simulink model "plateforme_seule_matlab"  (R2016a)
settings: Solver=VariableStepAuto  StartTime=0.0  StopTime=10  RelTol=1e-3
model workspace: external: MATLAB File C:\Users\costa\Documents\Renaud\Dorian\Prepa\Studies\Carte aquisition Stewart\Matlab-SW\plateforme_seule_matlab_DataFile.m (data not in the file)
values from neighbouring files (symbols this model uses):
  K = 0.0135    [variables.m]
  Kd = 0    [variables.m]
  Ki = 0    [variables.m]
  Kp = 40    [variables.m]
  L0 = 380    [variables.m]
  R = 8.9    [variables.m]
undefined symbols (not defined in the file or in its folder): smiData, X, Y, Z
libraries: sm_lib x361, fl_lib x60, nesl_utility x13, simulink x6
(part 3 of 9)

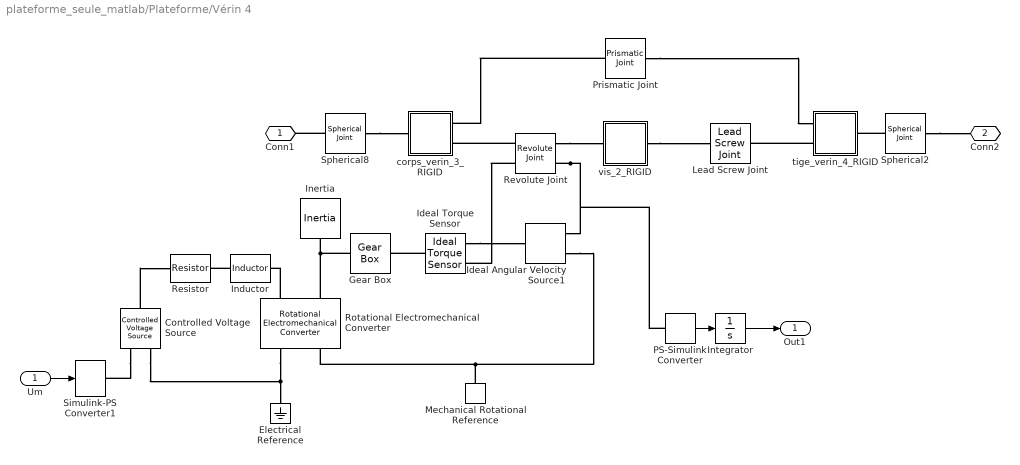
== system plateforme_seule_matlab/Plateforme/Vérin 4 ==
  Um : Inport
  Controlled Voltage Source : fl_lib/Electrical/Electrical Sources/Controlled Voltage Source
  Electrical Reference : fl_lib/Electrical/Electrical Elements/Electrical Reference
  Gear Box : fl_lib/Mechanical/Mechanisms/Gear Box  ratio=red  t_in_specify=off  t_in_priority=None  t_in=0 N*m  t_out_specify=off  t_out_priority=None  t_out=0 N*m
  Ideal Angular Velocity Source1 : fl_lib/Mechanical/Mechanical Sources/Ideal Angular Velocity Source
  Ideal Torque Sensor : fl_lib/Mechanical/Mechanical Sensors/Ideal Torque Sensor
  Inductor : fl_lib/Electrical/Electrical Elements/Inductor  l=L H  r=0 Ohm  g=1e-9 1/Ohm  i_specify=off  i_priority=None  i=0 A  v_specify=off  v_priority=None  v=0 V  i_L_specify=off  i_L_priority=High  i_L=0 A
  Inertia : fl_lib/Mechanical/Rotational Elements/Inertia  inertia=J kg*m^2  w_specify=off  w_priority=High  w=0 rad/s  t_specify=off  t_priority=None  t=0 N*m
  Integrator : Integrator  InitialCondition=L0
  Lead Screw Joint : sm_lib/Joints/Lead Screw Joint  SenseConstraintForce=off  SenseConstraintForceX=off  SenseConstraintForceY=off  SenseConstraintForceZ=off  SenseConstraintTorque=off  SenseConstraintTorqueX=off  SenseConstraintTorqueY=off  SenseConstraintTorqueZ=off  SenseTotalForce=off  SenseTotalForceX=off  SenseTotalForceY=off  SenseTotalForceZ=off  SenseTotalTorque=off  SenseTotalTorqueX=off  SenseTotalTorqueY=off  SenseTotalTorqueZ=off  CompositeWrenchDir=FollowerOnBase  CompositeWrenchFrame=BaseFrame  Direction=RightHand  Lead=6.35  LeadUnits=mm/rev  SenseRotationPosition=off  SenseRotationVelocity=off  SenseRotationAcceleration=off  SenseTranslationPosition=off  SenseTranslationVelocity=off  SenseTranslationAcceleration=off  PositionTargetSpecify=off  PositionTargetPriority=High  PositionTargetRotationBased=off  PositionTargetRotationValue=0  PositionTargetRotationValueUnits=deg  PositionTargetTranslationValue=0  PositionTargetTranslationValueUnits=m  VelocityTargetSpecify=off  VelocityTargetPriority=High  VelocityTargetRotationBased=off  VelocityTargetRotationValue=0  VelocityTargetRotationValueUnits=deg/s  VelocityTargetTranslationValue=0  VelocityTargetTranslationValueUnits=m/s
  Mechanical Rotational Reference : fl_lib/Mechanical/Rotational Elements/Mechanical Rotational Reference
  PS-Simulink Converter : nesl_utility/PS-Simulink Converter  PhysicalDomain=network_engine_domain  SubClassName=ps_output  LeftPortType=input  RightPortType=output  PseudoPeriodic=off  Frequencies=[]  Unit=rad/s  AffineConversion=off
  Prismatic Joint : sm_lib/Joints/Prismatic Joint  SenseConstraintForce=off  SenseConstraintForceX=off  SenseConstraintForceY=off  SenseConstraintForceZ=off  SenseConstraintTorque=off  SenseConstraintTorqueX=off  SenseConstraintTorqueY=off  SenseConstraintTorqueZ=off  SenseTotalForce=off  SenseTotalForceX=off  SenseTotalForceY=off  SenseTotalForceZ=off  SenseTotalTorque=off  SenseTotalTorqueX=off  SenseTotalTorqueY=off  SenseTotalTorqueZ=off  CompositeWrenchDir=FollowerOnBase  CompositeWrenchFrame=BaseFrame  EquilibriumPosition=L0  EquilibriumPositionUnits=m  SpringStiffness=0  SpringStiffnessUnits=N/m  DampingCoefficient=0  DampingCoefficientUnits=N/(m/s)  TorqueActuationMode=NoTorque  MotionActuationMode=ComputedMotion  SensePosition=off  SenseVelocity=off  SenseAcceleration=off  SenseTorqueForce=off  PositionTargetSpecify=off  PositionTargetPriority=High  PositionTargetValue=L0  PositionTargetValueUnits=m  VelocityTargetSpecify=off  VelocityTargetPriority=High  VelocityTargetValue=0  VelocityTargetValueUnits=m/s
  Resistor : fl_lib/Electrical/Electrical Elements/Resistor  R=R Ohm  i_specify=off  i_priority=None  i=0 A  v_specify=off  v_priority=None  v=0 V
  Revolute Joint : sm_lib/Joints/Revolute Joint  SenseConstraintForce=off  SenseConstraintForceX=off  SenseConstraintForceY=off  SenseConstraintForceZ=off  SenseConstraintTorque=off  SenseConstraintTorqueX=off  SenseConstraintTorqueY=off  SenseConstraintTorqueZ=off  SenseTotalForce=off  SenseTotalForceX=off  SenseTotalForceY=off  SenseTotalForceZ=off  SenseTotalTorque=off  SenseTotalTorqueX=off  SenseTotalTorqueY=off  SenseTotalTorqueZ=off  CompositeWrenchDir=FollowerOnBase  CompositeWrenchFrame=BaseFrame  EquilibriumPosition=0  EquilibriumPositionUnits=deg  SpringStiffness=0  SpringStiffnessUnits=N*m/deg  DampingCoefficient=0  DampingCoefficientUnits=N*m/(deg/s)  TorqueActuationMode=InputTorque  MotionActuationMode=ComputedMotion  SensePosition=off  SenseVelocity=on  SenseAcceleration=off  SenseTorqueForce=off  PositionTargetSpecify=off  PositionTargetPriority=High  PositionTargetValue=0  PositionTargetValueUnits=deg  VelocityTargetSpecify=off  VelocityTargetPriority=High  VelocityTargetValue=0  VelocityTargetValueUnits=deg/s
  Rotational Electromechanical Converter : fl_lib/Electrical/Electrical Elements/Rotational Electromechanical Converter  K=K V/(rad/s)  i_specify=off  i_priority=None  i=0 A  v_specify=off  v_priority=None  v=0 V  t_specify=off  t_priority=None  t=0 N*m  w_specify=off  w_priority=None  w=0 rad/s
  Simulink-PS Converter1 : nesl_utility/Simulink-PS Converter  PhysicalDomain=network_engine_domain  SubClassName=ps_input  LeftPortType=input  RightPortType=output  PseudoPeriodic=off  Frequencies=[]  NoiseDistribution=none  NoiseParameters=[]  Unit=V  AffineConversion=off  InputFiltering=off  SimscapeFilterOrder=1  InputFilterTimeConstant=0.001  UdotUserProvided=1
  Spherical2 : sm_lib/Joints/Spherical Joint  SenseConstraintForce=off  SenseConstraintForceX=off  SenseConstraintForceY=off  SenseConstraintForceZ=off  SenseConstraintTorque=off  SenseConstraintTorqueX=off  SenseConstraintTorqueY=off  SenseConstraintTorqueZ=off  SenseTotalForce=off  SenseTotalForceX=off  SenseTotalForceY=off  SenseTotalForceZ=off  SenseTotalTorque=off  SenseTotalTorqueX=off  SenseTotalTorqueY=off  SenseTotalTorqueZ=off  CompositeWrenchDir=FollowerOnBase  CompositeWrenchFrame=BaseFrame  DefPosRotationMethod=None  DefPosRotationAngleUnits=deg  DefPosRotationStandardAxis=+Z  DefPosRotationAngle=0.0  DefPosRotationArbitraryAxis=[0 0 1]  DefPosFollAlignAxisA=+X  DefPosBaseAlignAxisA=+Y  DefPosFollAlignAxisB=+Y  DefPosBaseAlignAxisB=+Z  DefPosRotationSequenceAxes=FollowerAxes  DefPosRotationSequence=XYX  DefPosRotationSequenceAngles=[0 0 0]  DefPosRotationSequenceAnglesUnits=deg  DefPosRotationMatrix=[1 0 0; 0 1 0; 0 0 1]  EqPosRotationMethod=None  EqPosRotationAngleUnits=deg  EqPosRotationStandardAxis=+Z  EqPosRotationAngle=0.0  EqPosRotationArbitraryAxis=[0 0 1]  EqPosFollAlignAxisA=+X  EqPosBaseAlignAxisA=+Y  EqPosFollAlignAxisB=+Y  EqPosBaseAlignAxisB=+Z  EqPosRotationSequenceAxes=FollowerAxes  EqPosRotationSequence=XYX  EqPosRotationSequenceAngles=[0 0 0]  EqPosRotationSequenceAnglesUnits=deg  EqPosRotationMatrix=[1 0 0; 0 1 0; 0 0 1]  SpringStiffness=0  SpringStiffnessUnits=m*N/rad  DampingCoefficient=0  DampingCoefficientUnits=m*s*N/rad  ActuateTorqueX=off  ActuateTorqueY=off  ActuateTorqueZ=off  ActuateTorque=off  TorqueActuationMode=NoTorque  MotionActuationMode=ComputedMotion  ActuationFrame=BaseFrame  SensePosition=off  SenseVelocityX=off  SenseVelocityY=off  SenseVelocityZ=off  SenseVelocity=off  SenseAccelerationX=off  SenseAccelerationY=off  SenseAccelerationZ=off  SenseAcceleration=off  SenseTorqueX=off  SenseTorqueY=off  SenseTorqueZ=off  SenseTorqueForce=off  SensingFrame=FollowerFrame  PositionTargetRotationMethod=None  PositionTargetRotationAngleUnits=deg  PositionTargetRotationStandardAxis=+Z  PositionTargetRotationAngle=0.0  PositionTargetRotationArbitraryAxis=[0 0 1]  PositionTargetFollAlignAxisA=+X  PositionTargetBaseAlignAxisA=+Y  PositionTargetFollAlignAxisB=+Y  PositionTargetBaseAlignAxisB=+Z  PositionTargetRotationSequenceAxes=FollowerAxes  PositionTargetRotationSequence=XYX  PositionTargetRotationSequenceAngles=[0 0 0]  PositionTargetRotationSequenceAnglesUnits=deg  PositionTargetRotationMatrix=[1 0 0; 0 1 0; 0 0 1]  PositionTargetSpecify=off  PositionTargetPriority=High  VelocityTargetValue=[0 0 0]  VelocityTargetValueUnits=deg/s  VelocityTargetSpecify=off  VelocityTargetPriority=High  VelocityTargetInFollowerFrame=on
  Spherical8 : sm_lib/Joints/Spherical Joint  SenseConstraintForce=off  SenseConstraintForceX=off  SenseConstraintForceY=off  SenseConstraintForceZ=off  SenseConstraintTorque=off  SenseConstraintTorqueX=off  SenseConstraintTorqueY=off  SenseConstraintTorqueZ=off  SenseTotalForce=off  SenseTotalForceX=off  SenseTotalForceY=off  SenseTotalForceZ=off  SenseTotalTorque=off  SenseTotalTorqueX=off  SenseTotalTorqueY=off  SenseTotalTorqueZ=off  CompositeWrenchDir=FollowerOnBase  CompositeWrenchFrame=BaseFrame  DefPosRotationMethod=None  DefPosRotationAngleUnits=deg  DefPosRotationStandardAxis=+Z  DefPosRotationAngle=0.0  DefPosRotationArbitraryAxis=[0 0 1]  DefPosFollAlignAxisA=+X  DefPosBaseAlignAxisA=+Y  DefPosFollAlignAxisB=+Y  DefPosBaseAlignAxisB=+Z  DefPosRotationSequenceAxes=FollowerAxes  DefPosRotationSequence=XYX  DefPosRotationSequenceAngles=[0 0 0]  DefPosRotationSequenceAnglesUnits=deg  DefPosRotationMatrix=[1 0 0; 0 1 0; 0 0 1]  EqPosRotationMethod=None  EqPosRotationAngleUnits=deg  EqPosRotationStandardAxis=+Z  EqPosRotationAngle=0.0  EqPosRotationArbitraryAxis=[0 0 1]  EqPosFollAlignAxisA=+X  EqPosBaseAlignAxisA=+Y  EqPosFollAlignAxisB=+Y  EqPosBaseAlignAxisB=+Z  EqPosRotationSequenceAxes=FollowerAxes  EqPosRotationSequence=XYX  EqPosRotationSequenceAngles=[0 0 0]  EqPosRotationSequenceAnglesUnits=deg  EqPosRotationMatrix=[1 0 0; 0 1 0; 0 0 1]  SpringStiffness=0  SpringStiffnessUnits=m*N/rad  DampingCoefficient=0  DampingCoefficientUnits=m*s*N/rad  ActuateTorqueX=off  ActuateTorqueY=off  ActuateTorqueZ=off  ActuateTorque=off  TorqueActuationMode=NoTorque  MotionActuationMode=ComputedMotion  ActuationFrame=BaseFrame  SensePosition=off  SenseVelocityX=off  SenseVelocityY=off  SenseVelocityZ=off  SenseVelocity=off  SenseAccelerationX=off  SenseAccelerationY=off  SenseAccelerationZ=off  SenseAcceleration=off  SenseTorqueX=off  SenseTorqueY=off  SenseTorqueZ=off  SenseTorqueForce=off  SensingFrame=FollowerFrame  PositionTargetRotationMethod=ArbitraryAxis  PositionTargetRotationAngleUnits=deg  PositionTargetRotationStandardAxis=+Z  PositionTargetRotationAngle=smiData.SphericalJoint(9).S.Pos.Angle  PositionTargetRotationArbitraryAxis=smiData.SphericalJoint(9).S.Pos.Axis  PositionTargetFollAlignAxisA=+X  PositionTargetBaseAlignAxisA=+Y  PositionTargetFollAlignAxisB=+Y  PositionTargetBaseAlignAxisB=+Z  PositionTargetRotationSequenceAxes=FollowerAxes  PositionTargetRotationSequence=XYX  PositionTargetRotationSequenceAngles=[0 0 0]  PositionTargetRotationSequenceAnglesUnits=deg  PositionTargetRotationMatrix=[1 0 0; 0 1 0; 0 0 1]  PositionTargetSpecify=off  PositionTargetPriority=Low  VelocityTargetValue=[0 0 0]  VelocityTargetValueUnits=deg/s  VelocityTargetSpecify=off  VelocityTargetPriority=High  VelocityTargetInFollowerFrame=on
  corps_verin_3_RIGID : Subsystem
  tige_verin_4_RIGID : Subsystem
  vis_2_RIGID : Subsystem
  Conn1 : PMIOPort  Port=1  Side=Left
  Conn2 : PMIOPort  Port=2  Side=Right
  Out1 : Outport
  wires:
  Um/1 -> Simulink-PS Converter1/1
  PS-Simulink Converter/1 -> Integrator/1
  Integrator/1 -> Out1/1
  connections:
  Spherical8/LConn1 -- Conn1/RConn1
  Spherical8/RConn1 -- corps_verin_3_RIGID/LConn1
  Spherical2/LConn1 -- tige_verin_4_RIGID/RConn1
  Spherical2/RConn1 -- Conn2/RConn1
  Prismatic Joint/LConn1 -- corps_verin_3_RIGID/RConn1
  Prismatic Joint/RConn1 -- tige_verin_4_RIGID/LConn1
  Revolute Joint/LConn1 -- corps_verin_3_RIGID/RConn2
  tige_verin_4_RIGID/LConn2 -- Lead Screw Joint/RConn1
  vis_2_RIGID/RConn1 -- Lead Screw Joint/LConn1
  Revolute Joint/RConn1 -- vis_2_RIGID/LConn1
  Ideal Angular Velocity Source1/RConn2 -- Mechanical Rotational Reference/LConn1 -- Rotational Electromechanical Converter/RConn2
  Rotational Electromechanical Converter/LConn2 -- Gear Box/LConn1 -- Inertia/LConn1
  Controlled Voltage Source/RConn2 -- Rotational Electromechanical Converter/RConn1 -- Electrical Reference/LConn1
  Revolute Joint/RConn2 -- PS-Simulink Converter/LConn1 -- Ideal Angular Velocity Source1/RConn1
  Rotational Electromechanical Converter/LConn1 -- Inductor/RConn1
  Inductor/LConn1 -- Resistor/RConn1
  Controlled Voltage Source/LConn1 -- Resistor/LConn1
  Ideal Torque Sensor/RConn1 -- Ideal Angular Velocity Source1/LConn1
  Revolute Joint/LConn2 -- Ideal Torque Sensor/RConn2
  Ideal Torque Sensor/LConn1 -- Gear Box/RConn1
  Controlled Voltage Source/RConn1 -- Simulink-PS Converter1/RConn1

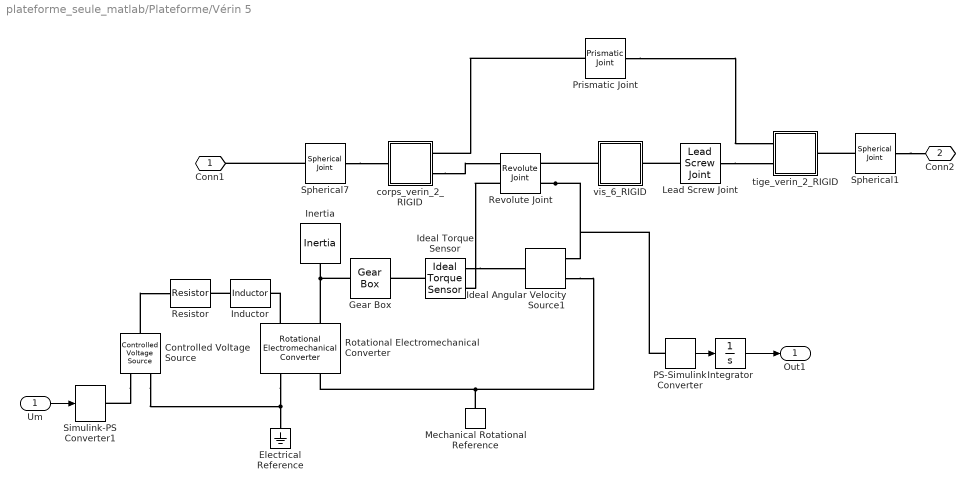
== system plateforme_seule_matlab/Plateforme/Vérin 5 ==
  Um : Inport
  Controlled Voltage Source : fl_lib/Electrical/Electrical Sources/Controlled Voltage Source
  Electrical Reference : fl_lib/Electrical/Electrical Elements/Electrical Reference
  Gear Box : fl_lib/Mechanical/Mechanisms/Gear Box  ratio=red  t_in_specify=off  t_in_priority=None  t_in=0 N*m  t_out_specify=off  t_out_priority=None  t_out=0 N*m
  Ideal Angular Velocity Source1 : fl_lib/Mechanical/Mechanical Sources/Ideal Angular Velocity Source
  Ideal Torque Sensor : fl_lib/Mechanical/Mechanical Sensors/Ideal Torque Sensor
  Inductor : fl_lib/Electrical/Electrical Elements/Inductor  l=L H  r=0 Ohm  g=1e-9 1/Ohm  i_specify=off  i_priority=None  i=0 A  v_specify=off  v_priority=None  v=0 V  i_L_specify=off  i_L_priority=High  i_L=0 A
  Inertia : fl_lib/Mechanical/Rotational Elements/Inertia  inertia=J kg*m^2  w_specify=off  w_priority=High  w=0 rad/s  t_specify=off  t_priority=None  t=0 N*m
  Integrator : Integrator  InitialCondition=L0
  Lead Screw Joint : sm_lib/Joints/Lead Screw Joint  SenseConstraintForce=off  SenseConstraintForceX=off  SenseConstraintForceY=off  SenseConstraintForceZ=off  SenseConstraintTorque=off  SenseConstraintTorqueX=off  SenseConstraintTorqueY=off  SenseConstraintTorqueZ=off  SenseTotalForce=off  SenseTotalForceX=off  SenseTotalForceY=off  SenseTotalForceZ=off  SenseTotalTorque=off  SenseTotalTorqueX=off  SenseTotalTorqueY=off  SenseTotalTorqueZ=off  CompositeWrenchDir=FollowerOnBase  CompositeWrenchFrame=BaseFrame  Direction=RightHand  Lead=6.35  LeadUnits=mm/rev  SenseRotationPosition=off  SenseRotationVelocity=off  SenseRotationAcceleration=off  SenseTranslationPosition=off  SenseTranslationVelocity=off  SenseTranslationAcceleration=off  PositionTargetSpecify=off  PositionTargetPriority=High  PositionTargetRotationBased=off  PositionTargetRotationValue=0  PositionTargetRotationValueUnits=deg  PositionTargetTranslationValue=0  PositionTargetTranslationValueUnits=m  VelocityTargetSpecify=off  VelocityTargetPriority=High  VelocityTargetRotationBased=off  VelocityTargetRotationValue=0  VelocityTargetRotationValueUnits=deg/s  VelocityTargetTranslationValue=0  VelocityTargetTranslationValueUnits=m/s
  Mechanical Rotational Reference : fl_lib/Mechanical/Rotational Elements/Mechanical Rotational Reference
  PS-Simulink Converter : nesl_utility/PS-Simulink Converter  PhysicalDomain=network_engine_domain  SubClassName=ps_output  LeftPortType=input  RightPortType=output  PseudoPeriodic=off  Frequencies=[]  Unit=rad/s  AffineConversion=off
  Prismatic Joint : sm_lib/Joints/Prismatic Joint  SenseConstraintForce=off  SenseConstraintForceX=off  SenseConstraintForceY=off  SenseConstraintForceZ=off  SenseConstraintTorque=off  SenseConstraintTorqueX=off  SenseConstraintTorqueY=off  SenseConstraintTorqueZ=off  SenseTotalForce=off  SenseTotalForceX=off  SenseTotalForceY=off  SenseTotalForceZ=off  SenseTotalTorque=off  SenseTotalTorqueX=off  SenseTotalTorqueY=off  SenseTotalTorqueZ=off  CompositeWrenchDir=FollowerOnBase  CompositeWrenchFrame=BaseFrame  EquilibriumPosition=L0  EquilibriumPositionUnits=m  SpringStiffness=0  SpringStiffnessUnits=N/m  DampingCoefficient=0  DampingCoefficientUnits=N/(m/s)  TorqueActuationMode=NoTorque  MotionActuationMode=ComputedMotion  SensePosition=off  SenseVelocity=off  SenseAcceleration=off  SenseTorqueForce=off  PositionTargetSpecify=off  PositionTargetPriority=High  PositionTargetValue=L0  PositionTargetValueUnits=m  VelocityTargetSpecify=off  VelocityTargetPriority=High  VelocityTargetValue=0  VelocityTargetValueUnits=m/s
  Resistor : fl_lib/Electrical/Electrical Elements/Resistor  R=R Ohm  i_specify=off  i_priority=None  i=0 A  v_specify=off  v_priority=None  v=0 V
  Revolute Joint : sm_lib/Joints/Revolute Joint  SenseConstraintForce=off  SenseConstraintForceX=off  SenseConstraintForceY=off  SenseConstraintForceZ=off  SenseConstraintTorque=off  SenseConstraintTorqueX=off  SenseConstraintTorqueY=off  SenseConstraintTorqueZ=off  SenseTotalForce=off  SenseTotalForceX=off  SenseTotalForceY=off  SenseTotalForceZ=off  SenseTotalTorque=off  SenseTotalTorqueX=off  SenseTotalTorqueY=off  SenseTotalTorqueZ=off  CompositeWrenchDir=FollowerOnBase  CompositeWrenchFrame=BaseFrame  EquilibriumPosition=0  EquilibriumPositionUnits=deg  SpringStiffness=0  SpringStiffnessUnits=N*m/deg  DampingCoefficient=0  DampingCoefficientUnits=N*m/(deg/s)  TorqueActuationMode=InputTorque  MotionActuationMode=ComputedMotion  SensePosition=off  SenseVelocity=on  SenseAcceleration=off  SenseTorqueForce=off  PositionTargetSpecify=off  PositionTargetPriority=High  PositionTargetValue=0  PositionTargetValueUnits=deg  VelocityTargetSpecify=off  VelocityTargetPriority=High  VelocityTargetValue=0  VelocityTargetValueUnits=deg/s
  Rotational Electromechanical Converter : fl_lib/Electrical/Electrical Elements/Rotational Electromechanical Converter  K=K V/(rad/s)  i_specify=off  i_priority=None  i=0 A  v_specify=off  v_priority=None  v=0 V  t_specify=off  t_priority=None  t=0 N*m  w_specify=off  w_priority=None  w=0 rad/s
  Simulink-PS Converter1 : nesl_utility/Simulink-PS Converter  PhysicalDomain=network_engine_domain  SubClassName=ps_input  LeftPortType=input  RightPortType=output  PseudoPeriodic=off  Frequencies=[]  NoiseDistribution=none  NoiseParameters=[]  Unit=V  AffineConversion=off  InputFiltering=off  SimscapeFilterOrder=1  InputFilterTimeConstant=0.001  UdotUserProvided=1
  Spherical1 : sm_lib/Joints/Spherical Joint  SenseConstraintForce=off  SenseConstraintForceX=off  SenseConstraintForceY=off  SenseConstraintForceZ=off  SenseConstraintTorque=off  SenseConstraintTorqueX=off  SenseConstraintTorqueY=off  SenseConstraintTorqueZ=off  SenseTotalForce=off  SenseTotalForceX=off  SenseTotalForceY=off  SenseTotalForceZ=off  SenseTotalTorque=off  SenseTotalTorqueX=off  SenseTotalTorqueY=off  SenseTotalTorqueZ=off  CompositeWrenchDir=FollowerOnBase  CompositeWrenchFrame=BaseFrame  DefPosRotationMethod=None  DefPosRotationAngleUnits=deg  DefPosRotationStandardAxis=+Z  DefPosRotationAngle=0.0  DefPosRotationArbitraryAxis=[0 0 1]  DefPosFollAlignAxisA=+X  DefPosBaseAlignAxisA=+Y  DefPosFollAlignAxisB=+Y  DefPosBaseAlignAxisB=+Z  DefPosRotationSequenceAxes=FollowerAxes  DefPosRotationSequence=XYX  DefPosRotationSequenceAngles=[0 0 0]  DefPosRotationSequenceAnglesUnits=deg  DefPosRotationMatrix=[1 0 0; 0 1 0; 0 0 1]  EqPosRotationMethod=None  EqPosRotationAngleUnits=deg  EqPosRotationStandardAxis=+Z  EqPosRotationAngle=0.0  EqPosRotationArbitraryAxis=[0 0 1]  EqPosFollAlignAxisA=+X  EqPosBaseAlignAxisA=+Y  EqPosFollAlignAxisB=+Y  EqPosBaseAlignAxisB=+Z  EqPosRotationSequenceAxes=FollowerAxes  EqPosRotationSequence=XYX  EqPosRotationSequenceAngles=[0 0 0]  EqPosRotationSequenceAnglesUnits=deg  EqPosRotationMatrix=[1 0 0; 0 1 0; 0 0 1]  SpringStiffness=0  SpringStiffnessUnits=m*N/rad  DampingCoefficient=0  DampingCoefficientUnits=m*s*N/rad  ActuateTorqueX=off  ActuateTorqueY=off  ActuateTorqueZ=off  ActuateTorque=off  TorqueActuationMode=NoTorque  MotionActuationMode=ComputedMotion  ActuationFrame=BaseFrame  SensePosition=off  SenseVelocityX=off  SenseVelocityY=off  SenseVelocityZ=off  SenseVelocity=off  SenseAccelerationX=off  SenseAccelerationY=off  SenseAccelerationZ=off  SenseAcceleration=off  SenseTorqueX=off  SenseTorqueY=off  SenseTorqueZ=off  SenseTorqueForce=off  SensingFrame=FollowerFrame  PositionTargetRotationMethod=None  PositionTargetRotationAngleUnits=deg  PositionTargetRotationStandardAxis=+Z  PositionTargetRotationAngle=0.0  PositionTargetRotationArbitraryAxis=[0 0 1]  PositionTargetFollAlignAxisA=+X  PositionTargetBaseAlignAxisA=+Y  PositionTargetFollAlignAxisB=+Y  PositionTargetBaseAlignAxisB=+Z  PositionTargetRotationSequenceAxes=FollowerAxes  PositionTargetRotationSequence=XYX  PositionTargetRotationSequenceAngles=[0 0 0]  PositionTargetRotationSequenceAnglesUnits=deg  PositionTargetRotationMatrix=[1 0 0; 0 1 0; 0 0 1]  PositionTargetSpecify=off  PositionTargetPriority=High  VelocityTargetValue=[0 0 0]  VelocityTargetValueUnits=deg/s  VelocityTargetSpecify=off  VelocityTargetPriority=High  VelocityTargetInFollowerFrame=on
  Spherical7 : sm_lib/Joints/Spherical Joint  SenseConstraintForce=off  SenseConstraintForceX=off  SenseConstraintForceY=off  SenseConstraintForceZ=off  SenseConstraintTorque=off  SenseConstraintTorqueX=off  SenseConstraintTorqueY=off  SenseConstraintTorqueZ=off  SenseTotalForce=off  SenseTotalForceX=off  SenseTotalForceY=off  SenseTotalForceZ=off  SenseTotalTorque=off  SenseTotalTorqueX=off  SenseTotalTorqueY=off  SenseTotalTorqueZ=off  CompositeWrenchDir=FollowerOnBase  CompositeWrenchFrame=BaseFrame  DefPosRotationMethod=None  DefPosRotationAngleUnits=deg  DefPosRotationStandardAxis=+Z  DefPosRotationAngle=0.0  DefPosRotationArbitraryAxis=[0 0 1]  DefPosFollAlignAxisA=+X  DefPosBaseAlignAxisA=+Y  DefPosFollAlignAxisB=+Y  DefPosBaseAlignAxisB=+Z  DefPosRotationSequenceAxes=FollowerAxes  DefPosRotationSequence=XYX  DefPosRotationSequenceAngles=[0 0 0]  DefPosRotationSequenceAnglesUnits=deg  DefPosRotationMatrix=[1 0 0; 0 1 0; 0 0 1]  EqPosRotationMethod=None  EqPosRotationAngleUnits=deg  EqPosRotationStandardAxis=+Z  EqPosRotationAngle=0.0  EqPosRotationArbitraryAxis=[0 0 1]  EqPosFollAlignAxisA=+X  EqPosBaseAlignAxisA=+Y  EqPosFollAlignAxisB=+Y  EqPosBaseAlignAxisB=+Z  EqPosRotationSequenceAxes=FollowerAxes  EqPosRotationSequence=XYX  EqPosRotationSequenceAngles=[0 0 0]  EqPosRotationSequenceAnglesUnits=deg  EqPosRotationMatrix=[1 0 0; 0 1 0; 0 0 1]  SpringStiffness=0  SpringStiffnessUnits=m*N/rad  DampingCoefficient=0  DampingCoefficientUnits=m*s*N/rad  ActuateTorqueX=off  ActuateTorqueY=off  ActuateTorqueZ=off  ActuateTorque=off  TorqueActuationMode=NoTorque  MotionActuationMode=ComputedMotion  ActuationFrame=BaseFrame  SensePosition=off  SenseVelocityX=off  SenseVelocityY=off  SenseVelocityZ=off  SenseVelocity=off  SenseAccelerationX=off  SenseAccelerationY=off  SenseAccelerationZ=off  SenseAcceleration=off  SenseTorqueX=off  SenseTorqueY=off  SenseTorqueZ=off  SenseTorqueForce=off  SensingFrame=FollowerFrame  PositionTargetRotationMethod=ArbitraryAxis  PositionTargetRotationAngleUnits=deg  PositionTargetRotationStandardAxis=+Z  PositionTargetRotationAngle=smiData.SphericalJoint(8).S.Pos.Angle  PositionTargetRotationArbitraryAxis=smiData.SphericalJoint(8).S.Pos.Axis  PositionTargetFollAlignAxisA=+X  PositionTargetBaseAlignAxisA=+Y  PositionTargetFollAlignAxisB=+Y  PositionTargetBaseAlignAxisB=+Z  PositionTargetRotationSequenceAxes=FollowerAxes  PositionTargetRotationSequence=XYX  PositionTargetRotationSequenceAngles=[0 0 0]  PositionTargetRotationSequenceAnglesUnits=deg  PositionTargetRotationMatrix=[1 0 0; 0 1 0; 0 0 1]  PositionTargetSpecify=off  PositionTargetPriority=Low  VelocityTargetValue=[0 0 0]  VelocityTargetValueUnits=deg/s  VelocityTargetSpecify=off  VelocityTargetPriority=High  VelocityTargetInFollowerFrame=on
  corps_verin_2_RIGID : Subsystem
  tige_verin_2_RIGID : Subsystem
  vis_6_RIGID : Subsystem
  Conn1 : PMIOPort  Port=1  Side=Left
  Conn2 : PMIOPort  Port=2  Side=Right
  Out1 : Outport
  wires:
  Um/1 -> Simulink-PS Converter1/1
  PS-Simulink Converter/1 -> Integrator/1
  Integrator/1 -> Out1/1
  connections:
  Spherical7/LConn1 -- Conn1/RConn1
  Lead Screw Joint/RConn1 -- tige_verin_2_RIGID/LConn2
  corps_verin_2_RIGID/RConn2 -- Revolute Joint/LConn1
  Lead Screw Joint/LConn1 -- vis_6_RIGID/RConn1
  Spherical7/RConn1 -- corps_verin_2_RIGID/LConn1
  Spherical1/LConn1 -- tige_verin_2_RIGID/RConn1
  vis_6_RIGID/LConn1 -- Revolute Joint/RConn1
  Spherical1/RConn1 -- Conn2/RConn1
  Prismatic Joint/RConn1 -- tige_verin_2_RIGID/LConn1
  Prismatic Joint/LConn1 -- corps_verin_2_RIGID/RConn1
  Ideal Angular Velocity Source1/RConn2 -- Mechanical Rotational Reference/LConn1 -- Rotational Electromechanical Converter/RConn2
  Rotational Electromechanical Converter/LConn2 -- Gear Box/LConn1 -- Inertia/LConn1
  Controlled Voltage Source/RConn2 -- Rotational Electromechanical Converter/RConn1 -- Electrical Reference/LConn1
  Revolute Joint/RConn2 -- Ideal Angular Velocity Source1/RConn1 -- PS-Simulink Converter/LConn1
  Rotational Electromechanical Converter/LConn1 -- Inductor/RConn1
  Inductor/LConn1 -- Resistor/RConn1
  Controlled Voltage Source/LConn1 -- Resistor/LConn1
  Ideal Torque Sensor/RConn1 -- Ideal Angular Velocity Source1/LConn1
  Revolute Joint/LConn2 -- Ideal Torque Sensor/RConn2
  Ideal Torque Sensor/LConn1 -- Gear Box/RConn1
  Controlled Voltage Source/RConn1 -- Simulink-PS Converter1/RConn1

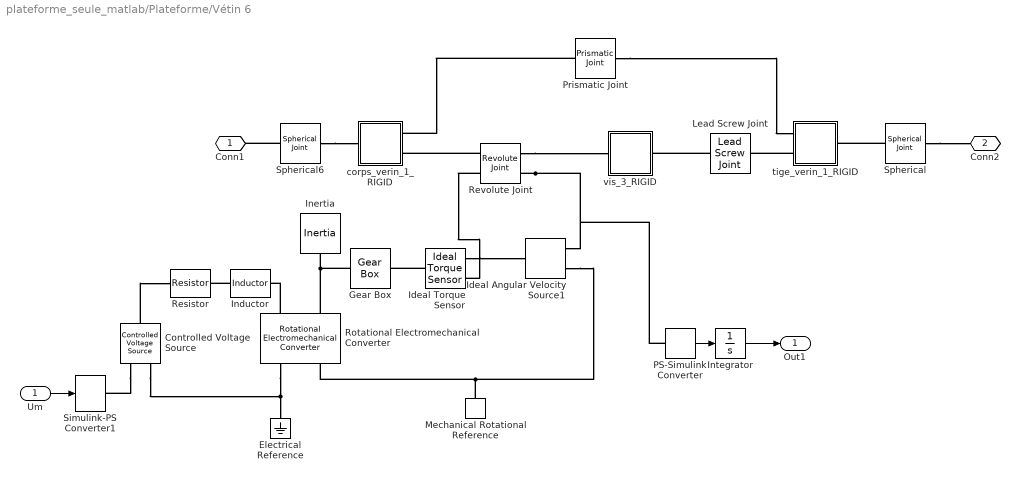
== system plateforme_seule_matlab/Plateforme/Vétin 6 ==
  Um : Inport
  Controlled Voltage Source : fl_lib/Electrical/Electrical Sources/Controlled Voltage Source
  Electrical Reference : fl_lib/Electrical/Electrical Elements/Electrical Reference
  Gear Box : fl_lib/Mechanical/Mechanisms/Gear Box  ratio=red  t_in_specify=off  t_in_priority=None  t_in=0 N*m  t_out_specify=off  t_out_priority=None  t_out=0 N*m
  Ideal Angular Velocity Source1 : fl_lib/Mechanical/Mechanical Sources/Ideal Angular Velocity Source
  Ideal Torque Sensor : fl_lib/Mechanical/Mechanical Sensors/Ideal Torque Sensor
  Inductor : fl_lib/Electrical/Electrical Elements/Inductor  l=L H  r=0 Ohm  g=1e-9 1/Ohm  i_specify=off  i_priority=None  i=0 A  v_specify=off  v_priority=None  v=0 V  i_L_specify=off  i_L_priority=High  i_L=0 A
  Inertia : fl_lib/Mechanical/Rotational Elements/Inertia  inertia=J kg*m^2  w_specify=off  w_priority=High  w=0 rad/s  t_specify=off  t_priority=None  t=0 N*m
  Integrator : Integrator  InitialCondition=L0
  Lead Screw Joint : sm_lib/Joints/Lead Screw Joint  SenseConstraintForce=off  SenseConstraintForceX=off  SenseConstraintForceY=off  SenseConstraintForceZ=off  SenseConstraintTorque=off  SenseConstraintTorqueX=off  SenseConstraintTorqueY=off  SenseConstraintTorqueZ=off  SenseTotalForce=off  SenseTotalForceX=off  SenseTotalForceY=off  SenseTotalForceZ=off  SenseTotalTorque=off  SenseTotalTorqueX=off  SenseTotalTorqueY=off  SenseTotalTorqueZ=off  CompositeWrenchDir=FollowerOnBase  CompositeWrenchFrame=BaseFrame  Direction=RightHand  Lead=6.35  LeadUnits=mm/rev  SenseRotationPosition=off  SenseRotationVelocity=off  SenseRotationAcceleration=off  SenseTranslationPosition=off  SenseTranslationVelocity=off  SenseTranslationAcceleration=off  PositionTargetSpecify=off  PositionTargetPriority=High  PositionTargetRotationBased=off  PositionTargetRotationValue=0  PositionTargetRotationValueUnits=deg  PositionTargetTranslationValue=0  PositionTargetTranslationValueUnits=m  VelocityTargetSpecify=off  VelocityTargetPriority=High  VelocityTargetRotationBased=off  VelocityTargetRotationValue=0  VelocityTargetRotationValueUnits=deg/s  VelocityTargetTranslationValue=0  VelocityTargetTranslationValueUnits=m/s
  Mechanical Rotational Reference : fl_lib/Mechanical/Rotational Elements/Mechanical Rotational Reference
  PS-Simulink Converter : nesl_utility/PS-Simulink Converter  PhysicalDomain=network_engine_domain  SubClassName=ps_output  LeftPortType=input  RightPortType=output  PseudoPeriodic=off  Frequencies=[]  Unit=rad/s  AffineConversion=off
  Prismatic Joint : sm_lib/Joints/Prismatic Joint  SenseConstraintForce=off  SenseConstraintForceX=off  SenseConstraintForceY=off  SenseConstraintForceZ=off  SenseConstraintTorque=off  SenseConstraintTorqueX=off  SenseConstraintTorqueY=off  SenseConstraintTorqueZ=off  SenseTotalForce=off  SenseTotalForceX=off  SenseTotalForceY=off  SenseTotalForceZ=off  SenseTotalTorque=off  SenseTotalTorqueX=off  SenseTotalTorqueY=off  SenseTotalTorqueZ=off  CompositeWrenchDir=FollowerOnBase  CompositeWrenchFrame=BaseFrame  EquilibriumPosition=L0  EquilibriumPositionUnits=m  SpringStiffness=0  SpringStiffnessUnits=N/m  DampingCoefficient=0  DampingCoefficientUnits=N/(m/s)  TorqueActuationMode=NoTorque  MotionActuationMode=ComputedMotion  SensePosition=off  SenseVelocity=off  SenseAcceleration=off  SenseTorqueForce=off  PositionTargetSpecify=off  PositionTargetPriority=High  PositionTargetValue=L0  PositionTargetValueUnits=m  VelocityTargetSpecify=off  VelocityTargetPriority=High  VelocityTargetValue=0  VelocityTargetValueUnits=m/s
  Resistor : fl_lib/Electrical/Electrical Elements/Resistor  R=R Ohm  i_specify=off  i_priority=None  i=0 A  v_specify=off  v_priority=None  v=0 V
  Revolute Joint : sm_lib/Joints/Revolute Joint  SenseConstraintForce=off  SenseConstraintForceX=off  SenseConstraintForceY=off  SenseConstraintForceZ=off  SenseConstraintTorque=off  SenseConstraintTorqueX=off  SenseConstraintTorqueY=off  SenseConstraintTorqueZ=off  SenseTotalForce=off  SenseTotalForceX=off  SenseTotalForceY=off  SenseTotalForceZ=off  SenseTotalTorque=off  SenseTotalTorqueX=off  SenseTotalTorqueY=off  SenseTotalTorqueZ=off  CompositeWrenchDir=FollowerOnBase  CompositeWrenchFrame=BaseFrame  EquilibriumPosition=0  EquilibriumPositionUnits=deg  SpringStiffness=0  SpringStiffnessUnits=N*m/deg  DampingCoefficient=0  DampingCoefficientUnits=N*m/(deg/s)  TorqueActuationMode=InputTorque  MotionActuationMode=ComputedMotion  SensePosition=off  SenseVelocity=on  SenseAcceleration=off  SenseTorqueForce=off  PositionTargetSpecify=off  PositionTargetPriority=High  PositionTargetValue=0  PositionTargetValueUnits=deg  VelocityTargetSpecify=off  VelocityTargetPriority=High  VelocityTargetValue=0  VelocityTargetValueUnits=deg/s
  Rotational Electromechanical Converter : fl_lib/Electrical/Electrical Elements/Rotational Electromechanical Converter  K=K V/(rad/s)  i_specify=off  i_priority=None  i=0 A  v_specify=off  v_priority=None  v=0 V  t_specify=off  t_priority=None  t=0 N*m  w_specify=off  w_priority=None  w=0 rad/s
  Simulink-PS Converter1 : nesl_utility/Simulink-PS Converter  PhysicalDomain=network_engine_domain  SubClassName=ps_input  LeftPortType=input  RightPortType=output  PseudoPeriodic=off  Frequencies=[]  NoiseDistribution=none  NoiseParameters=[]  Unit=V  AffineConversion=off  InputFiltering=off  SimscapeFilterOrder=1  InputFilterTimeConstant=0.001  UdotUserProvided=1
  Spherical : sm_lib/Joints/Spherical Joint  SenseConstraintForce=off  SenseConstraintForceX=off  SenseConstraintForceY=off  SenseConstraintForceZ=off  SenseConstraintTorque=off  SenseConstraintTorqueX=off  SenseConstraintTorqueY=off  SenseConstraintTorqueZ=off  SenseTotalForce=off  SenseTotalForceX=off  SenseTotalForceY=off  SenseTotalForceZ=off  SenseTotalTorque=off  SenseTotalTorqueX=off  SenseTotalTorqueY=off  SenseTotalTorqueZ=off  CompositeWrenchDir=FollowerOnBase  CompositeWrenchFrame=BaseFrame  DefPosRotationMethod=None  DefPosRotationAngleUnits=deg  DefPosRotationStandardAxis=+Z  DefPosRotationAngle=0.0  DefPosRotationArbitraryAxis=[0 0 1]  DefPosFollAlignAxisA=+X  DefPosBaseAlignAxisA=+Y  DefPosFollAlignAxisB=+Y  DefPosBaseAlignAxisB=+Z  DefPosRotationSequenceAxes=FollowerAxes  DefPosRotationSequence=XYX  DefPosRotationSequenceAngles=[0 0 0]  DefPosRotationSequenceAnglesUnits=deg  DefPosRotationMatrix=[1 0 0; 0 1 0; 0 0 1]  EqPosRotationMethod=None  EqPosRotationAngleUnits=deg  EqPosRotationStandardAxis=+Z  EqPosRotationAngle=0.0  EqPosRotationArbitraryAxis=[0 0 1]  EqPosFollAlignAxisA=+X  EqPosBaseAlignAxisA=+Y  EqPosFollAlignAxisB=+Y  EqPosBaseAlignAxisB=+Z  EqPosRotationSequenceAxes=FollowerAxes  EqPosRotationSequence=XYX  EqPosRotationSequenceAngles=[0 0 0]  EqPosRotationSequenceAnglesUnits=deg  EqPosRotationMatrix=[1 0 0; 0 1 0; 0 0 1]  SpringStiffness=0  SpringStiffnessUnits=m*N/rad  DampingCoefficient=0  DampingCoefficientUnits=m*s*N/rad  ActuateTorqueX=off  ActuateTorqueY=off  ActuateTorqueZ=off  ActuateTorque=off  TorqueActuationMode=NoTorque  MotionActuationMode=ComputedMotion  ActuationFrame=BaseFrame  SensePosition=off  SenseVelocityX=off  SenseVelocityY=off  SenseVelocityZ=off  SenseVelocity=off  SenseAccelerationX=off  SenseAccelerationY=off  SenseAccelerationZ=off  SenseAcceleration=off  SenseTorqueX=off  SenseTorqueY=off  SenseTorqueZ=off  SenseTorqueForce=off  SensingFrame=FollowerFrame  PositionTargetRotationMethod=ArbitraryAxis  PositionTargetRotationAngleUnits=deg  PositionTargetRotationStandardAxis=+Z  PositionTargetRotationAngle=smiData.SphericalJoint(1).S.Pos.Angle  PositionTargetRotationArbitraryAxis=smiData.SphericalJoint(1).S.Pos.Axis  PositionTargetFollAlignAxisA=+X  PositionTargetBaseAlignAxisA=+Y  PositionTargetFollAlignAxisB=+Y  PositionTargetBaseAlignAxisB=+Z  PositionTargetRotationSequenceAxes=FollowerAxes  PositionTargetRotationSequence=XYX  PositionTargetRotationSequenceAngles=[0 0 0]  PositionTargetRotationSequenceAnglesUnits=deg  PositionTargetRotationMatrix=[1 0 0; 0 1 0; 0 0 1]  PositionTargetSpecify=off  PositionTargetPriority=Low  VelocityTargetValue=[0 0 0]  VelocityTargetValueUnits=deg/s  VelocityTargetSpecify=off  VelocityTargetPriority=High  VelocityTargetInFollowerFrame=on
  Spherical6 : sm_lib/Joints/Spherical Joint  SenseConstraintForce=off  SenseConstraintForceX=off  SenseConstraintForceY=off  SenseConstraintForceZ=off  SenseConstraintTorque=off  SenseConstraintTorqueX=off  SenseConstraintTorqueY=off  SenseConstraintTorqueZ=off  SenseTotalForce=off  SenseTotalForceX=off  SenseTotalForceY=off  SenseTotalForceZ=off  SenseTotalTorque=off  SenseTotalTorqueX=off  SenseTotalTorqueY=off  SenseTotalTorqueZ=off  CompositeWrenchDir=FollowerOnBase  CompositeWrenchFrame=BaseFrame  DefPosRotationMethod=None  DefPosRotationAngleUnits=deg  DefPosRotationStandardAxis=+Z  DefPosRotationAngle=0.0  DefPosRotationArbitraryAxis=[0 0 1]  DefPosFollAlignAxisA=+X  DefPosBaseAlignAxisA=+Y  DefPosFollAlignAxisB=+Y  DefPosBaseAlignAxisB=+Z  DefPosRotationSequenceAxes=FollowerAxes  DefPosRotationSequence=XYX  DefPosRotationSequenceAngles=[0 0 0]  DefPosRotationSequenceAnglesUnits=deg  DefPosRotationMatrix=[1 0 0; 0 1 0; 0 0 1]  EqPosRotationMethod=None  EqPosRotationAngleUnits=deg  EqPosRotationStandardAxis=+Z  EqPosRotationAngle=0.0  EqPosRotationArbitraryAxis=[0 0 1]  EqPosFollAlignAxisA=+X  EqPosBaseAlignAxisA=+Y  EqPosFollAlignAxisB=+Y  EqPosBaseAlignAxisB=+Z  EqPosRotationSequenceAxes=FollowerAxes  EqPosRotationSequence=XYX  EqPosRotationSequenceAngles=[0 0 0]  EqPosRotationSequenceAnglesUnits=deg  EqPosRotationMatrix=[1 0 0; 0 1 0; 0 0 1]  SpringStiffness=0  SpringStiffnessUnits=m*N/rad  DampingCoefficient=0  DampingCoefficientUnits=m*s*N/rad  ActuateTorqueX=off  ActuateTorqueY=off  ActuateTorqueZ=off  ActuateTorque=off  TorqueActuationMode=NoTorque  MotionActuationMode=ComputedMotion  ActuationFrame=BaseFrame  SensePosition=off  SenseVelocityX=off  SenseVelocityY=off  SenseVelocityZ=off  SenseVelocity=off  SenseAccelerationX=off  SenseAccelerationY=off  SenseAccelerationZ=off  SenseAcceleration=off  SenseTorqueX=off  SenseTorqueY=off  SenseTorqueZ=off  SenseTorqueForce=off  SensingFrame=FollowerFrame  PositionTargetRotationMethod=ArbitraryAxis  PositionTargetRotationAngleUnits=deg  PositionTargetRotationStandardAxis=+Z  PositionTargetRotationAngle=smiData.SphericalJoint(7).S.Pos.Angle  PositionTargetRotationArbitraryAxis=smiData.SphericalJoint(7).S.Pos.Axis  PositionTargetFollAlignAxisA=+X  PositionTargetBaseAlignAxisA=+Y  PositionTargetFollAlignAxisB=+Y  PositionTargetBaseAlignAxisB=+Z  PositionTargetRotationSequenceAxes=FollowerAxes  PositionTargetRotationSequence=XYX  PositionTargetRotationSequenceAngles=[0 0 0]  PositionTargetRotationSequenceAnglesUnits=deg  PositionTargetRotationMatrix=[1 0 0; 0 1 0; 0 0 1]  PositionTargetSpecify=off  PositionTargetPriority=Low  VelocityTargetValue=[0 0 0]  VelocityTargetValueUnits=deg/s  VelocityTargetSpecify=off  VelocityTargetPriority=High  VelocityTargetInFollowerFrame=on
  corps_verin_1_RIGID : Subsystem
  tige_verin_1_RIGID : Subsystem
  vis_3_RIGID : Subsystem
  Conn1 : PMIOPort  Port=1  Side=Left
  Conn2 : PMIOPort  Port=2  Side=Right
  Out1 : Outport
  wires:
  Um/1 -> Simulink-PS Converter1/1
  PS-Simulink Converter/1 -> Integrator/1
  Integrator/1 -> Out1/1
  connections:
  Revolute Joint/RConn1 -- vis_3_RIGID/LConn1
  Lead Screw Joint/RConn1 -- vis_3_RIGID/RConn1
  Revolute Joint/LConn1 -- corps_verin_1_RIGID/RConn2
  Spherical6/RConn1 -- corps_verin_1_RIGID/LConn1
  Spherical/RConn1 -- Conn2/RConn1
  Spherical/LConn1 -- tige_verin_1_RIGID/RConn1
  Spherical6/LConn1 -- Conn1/RConn1
  tige_verin_1_RIGID/LConn2 -- Lead Screw Joint/LConn1
  Prismatic Joint/LConn1 -- corps_verin_1_RIGID/RConn1
  Prismatic Joint/RConn1 -- tige_verin_1_RIGID/LConn1
  Ideal Angular Velocity Source1/RConn2 -- Mechanical Rotational Reference/LConn1 -- Rotational Electromechanical Converter/RConn2
  Rotational Electromechanical Converter/LConn2 -- Gear Box/LConn1 -- Inertia/LConn1
  Controlled Voltage Source/RConn2 -- Rotational Electromechanical Converter/RConn1 -- Electrical Reference/LConn1
  Revolute Joint/RConn2 -- Ideal Angular Velocity Source1/RConn1 -- PS-Simulink Converter/LConn1
  Rotational Electromechanical Converter/LConn1 -- Inductor/RConn1
  Inductor/LConn1 -- Resistor/RConn1
  Controlled Voltage Source/LConn1 -- Resistor/LConn1
  Ideal Torque Sensor/RConn1 -- Ideal Angular Velocity Source1/LConn1
  Revolute Joint/LConn2 -- Ideal Torque Sensor/RConn2
  Ideal Torque Sensor/LConn1 -- Gear Box/RConn1
  Controlled Voltage Source/RConn1 -- Simulink-PS Converter1/RConn1

== system plateforme_seule_matlab/Plateforme/Embase/embase_1_RIGID ==
  ReferenceFrame : sm_lib/Frames and Transforms/Reference Frame
  Solid : sm_lib/Body Elements/Solid  InertiaType=Custom  Mass=smiData.Solid(14).mass  MassUnits=kg  CenterOfMass=smiData.Solid(14).CoM  CenterOfMassUnits=mm  MomentsOfInertia=smiData.Solid(14).MoI  MomentsOfInertiaUnits=kg*mm^2  ProductsOfInertia=smiData.Solid(14).PoI  ProductsOfInertiaUnits=kg*mm^2  DensityBased=on  Density=1000  DensityUnits=kg/(m^3)  DoExposeReferenceFrame=on  SerializedFrames=<Frames/>  GraphicType=FromGeometry  MarkerShape=Sphere  MarkerSize=10  GraphicVisPropType=SimpleVisualProperties  GraphicDiffuseColor=smiData.Solid(14).color  GraphicSpecularColor=[0.5 0.5 0.5 1.0]  GraphicAmbientColor=[0.15 0.15 0.15 1.0]  GraphicEmissiveColor=[0.0 0.0 0.0 1.0]  GraphicShininess=75  GraphicOpacity=smiData.Solid(14).opacity  GeometryShape=FromFile  RectangleSize=[1 1]  RectangleSizeUnits=m  BrickDimensions=[1 1 1]  BrickDimensionUnits=m  CylinderRadius=1  CylinderRadiusUnits=m  CylinderLength=1  CylinderLengthUnits=m  SphereRadius=1  SphereRadiusUnits=m  EllipsoidRadii=[1 1 1]  EllipsoidRadiiUnits=m  ExtrusionCrossSection=[1 1; -1 1; -1 -1; 1 -1]  ExtrusionCrossSectionUnits=m  ExtrusionLength=1  ExtrusionLengthUnits=m  PolygonNumSides=3  PolygonOuterRadius=1  PolygonOuterRadiusUnits=m  ExtGeomFileType=STEP  ExtGeomFileName=embase_Défaut_sldprt.STEP  ExtGeomFileUnits=m  RevolutionCrossSection=[1 1; 1 -1; 2 -1; 2 1]  RevolutionCrossSectionUnits=m  RevolutionExtent=Full  RevolutionAngle=180  RevolutionAngleUnits=deg
  F : PMIOPort  Port=1  Side=Left
  connections:
  Solid/RConn1 -- ReferenceFrame/RConn1 -- F/RConn1

== system plateforme_seule_matlab/Plateforme/Embase/ext_sph_1_RIGID ==
  ReferenceFrame : sm_lib/Frames and Transforms/Reference Frame
  Solid : sm_lib/Body Elements/Solid  InertiaType=Custom  Mass=smiData.Solid(9).mass  MassUnits=kg  CenterOfMass=smiData.Solid(9).CoM  CenterOfMassUnits=mm  MomentsOfInertia=smiData.Solid(9).MoI  MomentsOfInertiaUnits=kg*mm^2  ProductsOfInertia=smiData.Solid(9).PoI  ProductsOfInertiaUnits=kg*mm^2  DensityBased=on  Density=1000  DensityUnits=kg/(m^3)  DoExposeReferenceFrame=on  SerializedFrames=<Frames/>  GraphicType=FromGeometry  MarkerShape=Sphere  MarkerSize=10  GraphicVisPropType=SimpleVisualProperties  GraphicDiffuseColor=smiData.Solid(9).color  GraphicSpecularColor=[0.5 0.5 0.5 1.0]  GraphicAmbientColor=[0.15 0.15 0.15 1.0]  GraphicEmissiveColor=[0.0 0.0 0.0 1.0]  GraphicShininess=75  GraphicOpacity=smiData.Solid(9).opacity  GeometryShape=FromFile  RectangleSize=[1 1]  RectangleSizeUnits=m  BrickDimensions=[1 1 1]  BrickDimensionUnits=m  CylinderRadius=1  CylinderRadiusUnits=m  CylinderLength=1  CylinderLengthUnits=m  SphereRadius=1  SphereRadiusUnits=m  EllipsoidRadii=[1 1 1]  EllipsoidRadiiUnits=m  ExtrusionCrossSection=[1 1; -1 1; -1 -1; 1 -1]  ExtrusionCrossSectionUnits=m  ExtrusionLength=1  ExtrusionLengthUnits=m  PolygonNumSides=3  PolygonOuterRadius=1  PolygonOuterRadiusUnits=m  ExtGeomFileType=STEP  ExtGeomFileName=ext_sph_Défaut_sldprt.STEP  ExtGeomFileUnits=m  RevolutionCrossSection=[1 1; 1 -1; 2 -1; 2 1]  RevolutionCrossSectionUnits=m  RevolutionExtent=Full  RevolutionAngle=180  RevolutionAngleUnits=deg
  F : PMIOPort  Port=1  Side=Left
  connections:
  Solid/RConn1 -- ReferenceFrame/RConn1 -- F/RConn1

== system plateforme_seule_matlab/Plateforme/Embase/ext_sph_2_RIGID ==
  ReferenceFrame : sm_lib/Frames and Transforms/Reference Frame
  Solid : sm_lib/Body Elements/Solid  InertiaType=Custom  Mass=smiData.Solid(9).mass  MassUnits=kg  CenterOfMass=smiData.Solid(9).CoM  CenterOfMassUnits=mm  MomentsOfInertia=smiData.Solid(9).MoI  MomentsOfInertiaUnits=kg*mm^2  ProductsOfInertia=smiData.Solid(9).PoI  ProductsOfInertiaUnits=kg*mm^2  DensityBased=on  Density=1000  DensityUnits=kg/(m^3)  DoExposeReferenceFrame=on  SerializedFrames=<Frames/>  GraphicType=FromGeometry  MarkerShape=Sphere  MarkerSize=10  GraphicVisPropType=SimpleVisualProperties  GraphicDiffuseColor=smiData.Solid(9).color  GraphicSpecularColor=[0.5 0.5 0.5 1.0]  GraphicAmbientColor=[0.15 0.15 0.15 1.0]  GraphicEmissiveColor=[0.0 0.0 0.0 1.0]  GraphicShininess=75  GraphicOpacity=smiData.Solid(9).opacity  GeometryShape=FromFile  RectangleSize=[1 1]  RectangleSizeUnits=m  BrickDimensions=[1 1 1]  BrickDimensionUnits=m  CylinderRadius=1  CylinderRadiusUnits=m  CylinderLength=1  CylinderLengthUnits=m  SphereRadius=1  SphereRadiusUnits=m  EllipsoidRadii=[1 1 1]  EllipsoidRadiiUnits=m  ExtrusionCrossSection=[1 1; -1 1; -1 -1; 1 -1]  ExtrusionCrossSectionUnits=m  ExtrusionLength=1  ExtrusionLengthUnits=m  PolygonNumSides=3  PolygonOuterRadius=1  PolygonOuterRadiusUnits=m  ExtGeomFileType=STEP  ExtGeomFileName=ext_sph_Défaut_sldprt.STEP  ExtGeomFileUnits=m  RevolutionCrossSection=[1 1; 1 -1; 2 -1; 2 1]  RevolutionCrossSectionUnits=m  RevolutionExtent=Full  RevolutionAngle=180  RevolutionAngleUnits=deg
  F : PMIOPort  Port=1  Side=Left
  connections:
  Solid/RConn1 -- ReferenceFrame/RConn1 -- F/RConn1

== system plateforme_seule_matlab/Plateforme/Embase/ext_sph_3_RIGID ==
  ReferenceFrame : sm_lib/Frames and Transforms/Reference Frame
  Solid : sm_lib/Body Elements/Solid  InertiaType=Custom  Mass=smiData.Solid(9).mass  MassUnits=kg  CenterOfMass=smiData.Solid(9).CoM  CenterOfMassUnits=mm  MomentsOfInertia=smiData.Solid(9).MoI  MomentsOfInertiaUnits=kg*mm^2  ProductsOfInertia=smiData.Solid(9).PoI  ProductsOfInertiaUnits=kg*mm^2  DensityBased=on  Density=1000  DensityUnits=kg/(m^3)  DoExposeReferenceFrame=on  SerializedFrames=<Frames/>  GraphicType=FromGeometry  MarkerShape=Sphere  MarkerSize=10  GraphicVisPropType=SimpleVisualProperties  GraphicDiffuseColor=smiData.Solid(9).color  GraphicSpecularColor=[0.5 0.5 0.5 1.0]  GraphicAmbientColor=[0.15 0.15 0.15 1.0]  GraphicEmissiveColor=[0.0 0.0 0.0 1.0]  GraphicShininess=75  GraphicOpacity=smiData.Solid(9).opacity  GeometryShape=FromFile  RectangleSize=[1 1]  RectangleSizeUnits=m  BrickDimensions=[1 1 1]  BrickDimensionUnits=m  CylinderRadius=1  CylinderRadiusUnits=m  CylinderLength=1  CylinderLengthUnits=m  SphereRadius=1  SphereRadiusUnits=m  EllipsoidRadii=[1 1 1]  EllipsoidRadiiUnits=m  ExtrusionCrossSection=[1 1; -1 1; -1 -1; 1 -1]  ExtrusionCrossSectionUnits=m  ExtrusionLength=1  ExtrusionLengthUnits=m  PolygonNumSides=3  PolygonOuterRadius=1  PolygonOuterRadiusUnits=m  ExtGeomFileType=STEP  ExtGeomFileName=ext_sph_Défaut_sldprt.STEP  ExtGeomFileUnits=m  RevolutionCrossSection=[1 1; 1 -1; 2 -1; 2 1]  RevolutionCrossSectionUnits=m  RevolutionExtent=Full  RevolutionAngle=180  RevolutionAngleUnits=deg
  F : PMIOPort  Port=1  Side=Left
  connections:
  Solid/RConn1 -- ReferenceFrame/RConn1 -- F/RConn1

== system plateforme_seule_matlab/Plateforme/Embase/ext_sph_4_RIGID ==
  ReferenceFrame : sm_lib/Frames and Transforms/Reference Frame
  Solid : sm_lib/Body Elements/Solid  InertiaType=Custom  Mass=smiData.Solid(9).mass  MassUnits=kg  CenterOfMass=smiData.Solid(9).CoM  CenterOfMassUnits=mm  MomentsOfInertia=smiData.Solid(9).MoI  MomentsOfInertiaUnits=kg*mm^2  ProductsOfInertia=smiData.Solid(9).PoI  ProductsOfInertiaUnits=kg*mm^2  DensityBased=on  Density=1000  DensityUnits=kg/(m^3)  DoExposeReferenceFrame=on  SerializedFrames=<Frames/>  GraphicType=FromGeometry  MarkerShape=Sphere  MarkerSize=10  GraphicVisPropType=SimpleVisualProperties  GraphicDiffuseColor=smiData.Solid(9).color  GraphicSpecularColor=[0.5 0.5 0.5 1.0]  GraphicAmbientColor=[0.15 0.15 0.15 1.0]  GraphicEmissiveColor=[0.0 0.0 0.0 1.0]  GraphicShininess=75  GraphicOpacity=smiData.Solid(9).opacity  GeometryShape=FromFile  RectangleSize=[1 1]  RectangleSizeUnits=m  BrickDimensions=[1 1 1]  BrickDimensionUnits=m  CylinderRadius=1  CylinderRadiusUnits=m  CylinderLength=1  CylinderLengthUnits=m  SphereRadius=1  SphereRadiusUnits=m  EllipsoidRadii=[1 1 1]  EllipsoidRadiiUnits=m  ExtrusionCrossSection=[1 1; -1 1; -1 -1; 1 -1]  ExtrusionCrossSectionUnits=m  ExtrusionLength=1  ExtrusionLengthUnits=m  PolygonNumSides=3  PolygonOuterRadius=1  PolygonOuterRadiusUnits=m  ExtGeomFileType=STEP  ExtGeomFileName=ext_sph_Défaut_sldprt.STEP  ExtGeomFileUnits=m  RevolutionCrossSection=[1 1; 1 -1; 2 -1; 2 1]  RevolutionCrossSectionUnits=m  RevolutionExtent=Full  RevolutionAngle=180  RevolutionAngleUnits=deg
  F : PMIOPort  Port=1  Side=Left
  connections:
  Solid/RConn1 -- ReferenceFrame/RConn1 -- F/RConn1

== system plateforme_seule_matlab/Plateforme/Embase/ext_sph_5_RIGID ==
  ReferenceFrame : sm_lib/Frames and Transforms/Reference Frame
  Solid : sm_lib/Body Elements/Solid  InertiaType=Custom  Mass=smiData.Solid(9).mass  MassUnits=kg  CenterOfMass=smiData.Solid(9).CoM  CenterOfMassUnits=mm  MomentsOfInertia=smiData.Solid(9).MoI  MomentsOfInertiaUnits=kg*mm^2  ProductsOfInertia=smiData.Solid(9).PoI  ProductsOfInertiaUnits=kg*mm^2  DensityBased=on  Density=1000  DensityUnits=kg/(m^3)  DoExposeReferenceFrame=on  SerializedFrames=<Frames/>  GraphicType=FromGeometry  MarkerShape=Sphere  MarkerSize=10  GraphicVisPropType=SimpleVisualProperties  GraphicDiffuseColor=smiData.Solid(9).color  GraphicSpecularColor=[0.5 0.5 0.5 1.0]  GraphicAmbientColor=[0.15 0.15 0.15 1.0]  GraphicEmissiveColor=[0.0 0.0 0.0 1.0]  GraphicShininess=75  GraphicOpacity=smiData.Solid(9).opacity  GeometryShape=FromFile  RectangleSize=[1 1]  RectangleSizeUnits=m  BrickDimensions=[1 1 1]  BrickDimensionUnits=m  CylinderRadius=1  CylinderRadiusUnits=m  CylinderLength=1  CylinderLengthUnits=m  SphereRadius=1  SphereRadiusUnits=m  EllipsoidRadii=[1 1 1]  EllipsoidRadiiUnits=m  ExtrusionCrossSection=[1 1; -1 1; -1 -1; 1 -1]  ExtrusionCrossSectionUnits=m  ExtrusionLength=1  ExtrusionLengthUnits=m  PolygonNumSides=3  PolygonOuterRadius=1  PolygonOuterRadiusUnits=m  ExtGeomFileType=STEP  ExtGeomFileName=ext_sph_Défaut_sldprt.STEP  ExtGeomFileUnits=m  RevolutionCrossSection=[1 1; 1 -1; 2 -1; 2 1]  RevolutionCrossSectionUnits=m  RevolutionExtent=Full  RevolutionAngle=180  RevolutionAngleUnits=deg
  F : PMIOPort  Port=1  Side=Left
  connections:
  Solid/RConn1 -- ReferenceFrame/RConn1 -- F/RConn1
